simulink model "HardwareInteg_draft2"  (R2023a)
settings: Solver=VariableStepAuto  StartTime=0.0  StopTime=inf  FixedStep=0.01  RelTol=1e-3
model workspace (MAT data in the model file):
  D = 0
  I = 0
  N = 100
  P = 1
  setpoint = 1
undefined symbols (not defined in the file or in its folder): daq
libraries: simulink x4, dspstat3 x3, daqlib x2, slpidlib x2, checkpacklib x1, spsTriangleGeneratorLib x1
settings Model: Creator=Siril TD  LastModifiedBy=Siril TD
settings OptimizationCC: DefaultParameterBehavior=Inlined  EnhancedBackFolding=on  PassReuseOutputArgsThreshold=0  OptimizeBlockOrder=speed  DifferentSizesBufferReuse=on
settings DebuggingCC: ParameterTunabilityLossMsg=error
settings HardwareCC: TargetBitPerPointer=64  TargetBitPerSizeT=64  TargetBitPerPtrDiffT=64  TargetLongLongMode=on  TargetIntDivRoundTo=Zero  TargetEndianess=LittleEndian  TargetWordSize=64  TargetHWDeviceType=MATLAB Host  ProdEqTarget=off
settings SFSimCC: SimGenImportedTypeDefs=on  SimTargetLang=C++
settings RTWCC: GenCodeOnly=on
settings CodeAppCC: ForceParamTrailComments=on  MaxIdLength=63  OperatorAnnotations=on

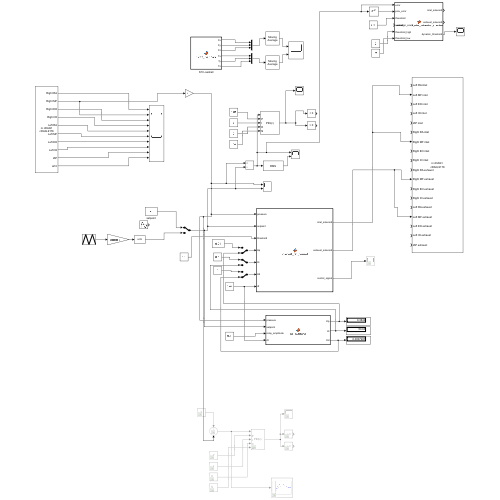
[thumbnail: Simulink's stored preview of the top-level diagram]
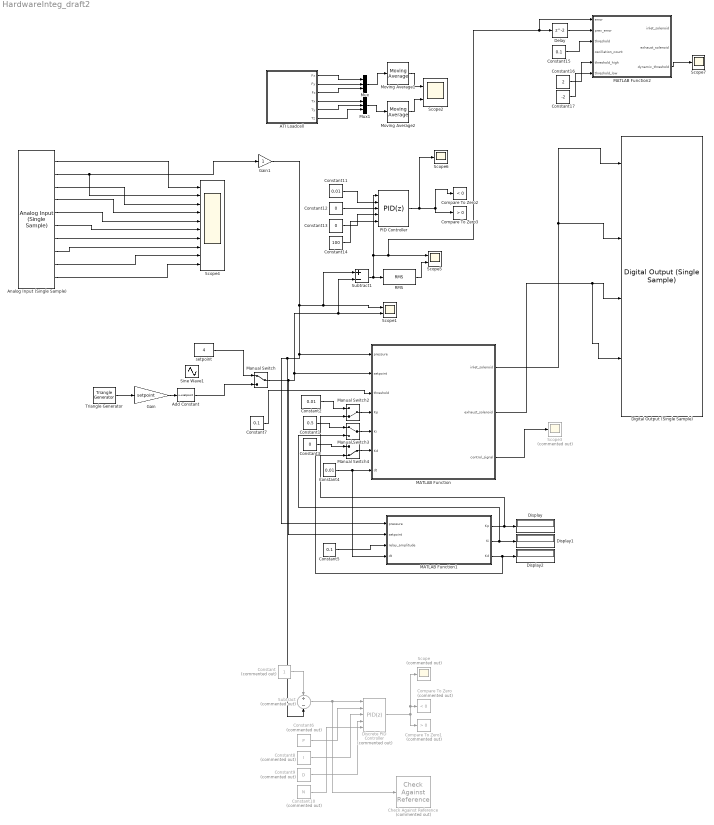
== system HardwareInteg_draft2 ==
  ATI Loadcell : MATLAB Function  TreatAsAtomicUnit=on
  Add Constant : Bias  Bias=setpoint  SaturateOnIntegerOverflow=off
  Analog Input (Single Sample) : daqlib/Analog Input (Single Sample)  DeviceMenu=ni cDAQ1 (cDAQ-9178)  Device=ni cDAQ1 (cDAQ-9178)  ModuleInfo=cDAQ1Mod1(NI 9205)  ObjConstructor=daq.createSession('ni')  BlockSampleTime=0.001  NChannelsSelected=10  Channels=0$ai0$$cDAQ1Mod1$1$4$1$1$#1$ai1$Right RA$cDAQ1Mod1$1$4$1$1$#1$ai2$Right MF$cDAQ1Mod1$1$4$1$1$#1$ai3$Right EO$cDAQ1Mod1$1$4$1$1$#1$ai4$Right IO$cDAQ1Mod1$1$4$1$1$#1$ai5$Left RA$cDAQ1Mod1$1$4$1$1$#1$ai6$Left MF$cDAQ1Mod1$1$4$1$1$#1$ai7$Left EO$cDAQ1Mod1$1$4$1$1$#1$ai8$Left IO$cDAQ1Mod1$1$4$1$1$#1$ai9$IAP$cDAQ1Mod1$1$4$1$1$#1$ai10$$cDAQ1Mod1$1$4$1$1$#0$ai11$$cDAQ1Mod1$1$4$1$1$#0$ai12$$cDAQ1Mod1$1$4$1$1$#0$ai13$$cDAQ1Mod1$1$4$1$1$#0$ai14$$cDAQ1Mod1$1$4$1$1$#0$ai15$$cDAQ1Mod1$1$4$1$1$#0$ai16$$cDAQ1Mod1$1$4$3$1$#0$ai17$$cDAQ1Mod1$1$4$3$1$#0$ai18$$cDAQ1Mod1$1$4$3$1$#0$ai19$$cDAQ1Mod1$1$4$3$1$#0$ai20$$cDAQ1Mod1$1$4$3$1$#0$ai21$$cDAQ1Mod1$1$4$3$1$#0$ai22$$cDAQ1Mod1$1$4$3$1$#0$ai23$$cDAQ1Mod1$1$4$3$1$#0$ai24$$cDAQ1Mod1$1$4$1$1$#0$ai25$$cDAQ1Mod1$1$4$1$1$#0$ai26$$cDAQ1Mod1$1$4$1$1$#0$ai27$$cDAQ1Mod1$1$4$1$1$#0$ai28$$cDAQ1Mod1$1$4$1$1$#0$ai29$$cDAQ1Mod1$1$4$1$1$#0$ai30$$cDAQ1Mod1$1$4$1$1$#0$ai31$$cDAQ1Mod1$1$4$1$1$#  NPorts=1 per channel  OutputTimestamp=off
  Check Against Reference : checkpacklib/Check Against Reference  Commented=on  InstantiateOnLoad=on  enabled=on  stopWhenAssertionFail=off  export=off  ViewDlgPos=[100 200 510 390]  OpenViewOnLoad=off  LaunchViewOnOpen=on  TimeUnits=seconds  EnableReferenceBound=on  AbsTolerance=0  RelTolerance=0.01  ReferenceTimes=[0 10]  ReferenceAmplitudes=[0 0]
      settings: LibrarySourceBlock=sdolib/Signal Constraints/Check Against Reference
  Compare To Zero : simulink/Logic and Bit Operations/Compare To Zero  Commented=on  relop=<  OutDataTypeStr=boolean
  Compare To Zero1 : simulink/Logic and Bit Operations/Compare To Zero  Commented=on  relop=>  OutDataTypeStr=boolean
  Compare To Zero2 : simulink/Logic and Bit Operations/Compare To Zero  relop=<  OutDataTypeStr=boolean
  Compare To Zero3 : simulink/Logic and Bit Operations/Compare To Zero  relop=>  OutDataTypeStr=boolean
  Constant : Constant  Commented=on
  Constant1 : Constant  Value=0.5
  Constant10 : Constant  Commented=on  Value=N
  Constant11 : Constant  Value=0.01
  Constant12 : Constant  Value=0
  Constant13 : Constant  Value=0
  Constant14 : Constant  Value=100
  Constant15 : Constant  Value=0.1
  Constant16 : Constant  Value=2
  Constant17 : Constant  Value=-2
  Constant2 : Constant  Value=0.01
  Constant3 : Constant  Value=0
  Constant4 : Constant  Value=0.01
  Constant5 : Constant  Value=0.1
  Constant6 : Constant  Commented=on  Value=P
  Constant7 : Constant  Value=0.1
  Constant8 : Constant  Commented=on  Value=I
  Constant9 : Constant  Commented=on  Value=D
  Delay : Delay
  Digital Output (Single Sample) : daqlib/Digital Output (Single Sample)  DeviceMenu=ni cDAQ1 (cDAQ-9178)  Device=ni cDAQ1 (cDAQ-9178)  ModuleInfo=cDAQ1Mod3(NI 9485)cDAQ1Mod4(NI 9485)cDAQ1Mod5(NI 9485)cDAQ1Mod6(NI 9485)  ObjConstructor=daq.createSession('ni')  BlockSampleTime=0.001  IsDigitalInput=off  NLinesSelected=18  Lines=0$port0/line0$$cDAQ1Mod3$#1$port0/line1$Left RA inlet$cDAQ1Mod3$#1$port0/line2$Left MF inlet$cDAQ1Mod3$#1$port0/line3$Left EO inlet$cDAQ1Mod3$#1$port0/line4$Left IO inlet$cDAQ1Mod3$#1$port0/line5$IAP inlet$cDAQ1Mod3$#0$port0/line6$$cDAQ1Mod3$#0$port0/line7$$cDAQ1Mod3$#0$port0/line0$$cDAQ1Mod4$#1$port0/line1$Right RA inlet$cDAQ1Mod4$#0$port0/line2$$cDAQ1Mod4$#1$port0/line3$Right MF inlet$cDAQ1Mod4$#0$port0/line4$$cDAQ1Mod4$#1$port0/line5$Right EO inlet$cDAQ1Mod4$#1$port0/line6$Right IO inlet$cDAQ1Mod4$#0$port0/line7$$cDAQ1Mod4$#0$port0/line0$$cDAQ1Mod5$#1$port0/line1$Right RA exhaust$cDAQ1Mod5$#0$port0/line2$$cDAQ1Mod5$#1$port0/line3$Right MF exhaust$cDAQ1Mod5$#0$port0/line4$$cDAQ1Mod5$#1$port0/line5$Right EO exhaust$cDAQ1Mod5$#1$port0/line6$Right IO exhaust$cDAQ1Mod5$#0$port0/line7$$cDAQ1Mod5$#0$port0/line0$$cDAQ1Mod6$#1$port0/line1$Left RA exhaust$cDAQ1Mod6$#1$port0/line2$Left MF exhaust$cDAQ1Mod6$#1$port0/line3$Left EO exhaust$cDAQ1Mod6$#1$port0/line4$Left IO exhaust$cDAQ1Mod6$#1$port0/line5$IAP exhaust$cDAQ1Mod6$#0$port0/line6$$cDAQ1Mod6$#0$port0/line7$$cDAQ1Mod6$#  NPorts=1 per line
  Discrete PID Controller : slpidlib/PID Controller  Commented=on  Controller=PID  Form=Parallel  TimeDomain=Discrete-time  UseExternalTs=off  SampleTime=0.01  IntegratorMethod=Forward Euler  FilterMethod=Forward Euler  ControllerParametersSource=external  P=0  I=-100  UseKiTs=off  D=0  N=100  UseFilter=on  TunerSelectOption=Transfer Function Based (PID Tuner App)  InitialConditionSource=internal  InitialConditionForIntegrator=0  InitialConditionForFilter=0  DifferentiatorICPrevScaledInput=0  ExternalReset=none  TrackingMode=off  Kt=1  LimitOutput=off  SatLimitsSource=internal  UpperSaturationLimit=inf  LowerSaturationLimit=-inf  LinearizeAsGain=off  AntiWindupMode=none  Kb=1  LimitIntegrator=off  UpperIntegratorSaturationLimit=inf  LowerIntegratorSaturationLimit=-inf  POutMin=[]  POutMax=[]  IOutMin=[]  IOutMax=[]  DOutMin=[]  DOutMax=[]  NOutMin=[]  NOutMax=[]  SumOutMin=[]  SumOutMax=[]  SaturationOutMin=[]  SaturationOutMax=[]  PParamMin=[]  PParamMax=[]  IParamMin=[]  IParamMax=[]  DParamMin=[]  DParamMax=[]  NParamMin=[]  NParamMax=[]  KbParamMin=[]  KbParamMax=[]  KtParamMin=[]  KtParamMax=[]  KbOutMin=[]  KbOutMax=[]  KtOutMin=[]  KtOutMax=[]  IntegratorOutMin=[]  IntegratorOutMax=[]  FilterOutMin=[]  FilterOutMax=[]  SumI1OutMin=[]  SumI1OutMax=[]  SumI2OutMin=[]  SumI2OutMax=[]  SumI3OutMin=[]  SumI3OutMax=[]  SumI4OutMin=[]  SumI4OutMax=[]  SumDOutMin=[]  SumDOutMax=[]  DifferentiatorOutMin=[]  DifferentiatorOutMax=[]  FilterDiffOutCoefMin=[]  FilterDiffOutCoefMax=[]  ReciprocalOutMin=[]  ReciprocalOutMax=[]  SumDenOutMin=[]  SumDenOutMax=[]  SumNumOutMin=[]  SumNumOutMax=[]  DivideOutMin=[]  DivideOutMax=[]  UdiffTsProdOutMin=[]  UdiffTsProdOutMax=[]  NTsProdOutMin=[]  NTsProdOutMax=[]  UintegralTsProdOutMin=[]  UintegralTsProdOutMax=[]  UngainTsProdOutMin=[]  UngainTsProdOutMax=[]  ClampingZeroOutDataTypeStr=Inherit: Inherit via back propagation  ClampingZeroOutMin=[]  ClampingZeroOutMax=[]  FilterDenConstantOutDataTypeStr=Inherit: Inherit via back propagation  FilterDenConstantOutMin=[]  FilterDenConstantOutMax=[]  PCopyOutDataTypeStr=Inherit: Inherit via back propagation  PCopyOutMin=[]  PCopyOutMax=[]  NCopyOutDataTypeStr=Inherit: Inherit via back propagation  NCopyOutMin=[]  NCopyOutMax=[]  IntegratorContinuousStateAttributes=''  IntegratorStateMustResolveToSignalObject=off  IntegratorRTWStateStorageClass=Auto  FilterContinuousStateAttributes=''  FilterStateMustResolveToSignalObject=off  FilterRTWStateStorageClass=Auto  ParallelPVariant=ExternalParameters  IdealPVariant=Disabled  IVariant=ExternalParameters  DVariant=ExternalParameters  IntegratorVariant=Discrete  SatVariant=Disabled  AWVariant=Passthrough  PCopyVariant=Disabled  TRVariant=Disabled  FdbkBlocksVariant=Forward  IdealPFdbkVariant=Disabled  SatFdbkVariant=Disabled  DerivativeFilterVariant=ForwardEulerFilter  NVariant=ExternalParameters  NCopyVariant=Disabled  FilterICVariant=InternalICsFilter  IntegratorICVariant=InternalICs  ExternalResetVariant=Disabled  TRSumVariant=Passthrough  SumFdbkVariant=Disabled  SumVariant=Sum_PID  TsampFilterVariant=InternalTs  TsampNgainVariant=Passthrough  TsampIntegralVariant=Disabled_SignalSpec  ExternalSaturationOutDataTypeStr=Inherit: Same as second input
      settings: LibrarySourceBlock=simulink/Discrete/Discrete PID Controller
  Display : Display
  Display1 : Display
  Display2 : Display
  Gain : Gain  Gain=setpoint
  Gain1 : Gain
  MATLAB Function : MATLAB Function  TreatAsAtomicUnit=on
  MATLAB Function1 : MATLAB Function  TreatAsAtomicUnit=on
  MATLAB Function2 : MATLAB Function  TreatAsAtomicUnit=on
  Manual Switch : ManualSwitch
  Manual Switch2 : ManualSwitch  CurrentSetting=0
  Manual Switch3 : ManualSwitch
  Manual Switch4 : ManualSwitch  CurrentSetting=0
  Moving Average1 : dspstat3/Moving Average  Method=Sliding window  ForgettingFactorPort=off  SpecifyWindowLength=on  WindowLength=4  OverlapLength=3  AllowArbitraryInputLength=off  ForgettingFactor=0.9  SimulateUsing=Code generation
  Moving Average2 : dspstat3/Moving Average  Method=Sliding window  ForgettingFactorPort=off  SpecifyWindowLength=on  WindowLength=4  OverlapLength=3  AllowArbitraryInputLength=off  ForgettingFactor=0.9  SimulateUsing=Code generation
  Mux : Mux  Inputs=3
  Mux1 : Mux  Inputs=3
  PID Controller : slpidlib/PID Controller  Controller=PID  Form=Parallel  TimeDomain=Discrete-time  UseExternalTs=off  SampleTime=-1  IntegratorMethod=Forward Euler  FilterMethod=Forward Euler  ControllerParametersSource=external  P=1  I=1  UseKiTs=off  D=0  N=100  UseFilter=on  TunerSelectOption=Transfer Function Based (PID Tuner App)  InitialConditionSource=internal  InitialConditionForIntegrator=0  InitialConditionForFilter=0  DifferentiatorICPrevScaledInput=0  ExternalReset=none  TrackingMode=off  Kt=1  LimitOutput=off  SatLimitsSource=internal  UpperSaturationLimit=inf  LowerSaturationLimit=-inf  LinearizeAsGain=on  AntiWindupMode=none  Kb=1  LimitIntegrator=off  UpperIntegratorSaturationLimit=inf  LowerIntegratorSaturationLimit=-inf  POutMin=[]  POutMax=[]  IOutMin=[]  IOutMax=[]  DOutMin=[]  DOutMax=[]  NOutMin=[]  NOutMax=[]  SumOutMin=[]  SumOutMax=[]  SaturationOutMin=[]  SaturationOutMax=[]  PParamMin=[]  PParamMax=[]  IParamMin=[]  IParamMax=[]  DParamMin=[]  DParamMax=[]  NParamMin=[]  NParamMax=[]  KbParamMin=[]  KbParamMax=[]  KtParamMin=[]  KtParamMax=[]  KbOutMin=[]  KbOutMax=[]  KtOutMin=[]  KtOutMax=[]  IntegratorOutMin=[]  IntegratorOutMax=[]  FilterOutMin=[]  FilterOutMax=[]  SumI1OutMin=[]  SumI1OutMax=[]  SumI2OutMin=[]  SumI2OutMax=[]  SumI3OutMin=[]  SumI3OutMax=[]  SumI4OutMin=[]  SumI4OutMax=[]  SumDOutMin=[]  SumDOutMax=[]  DifferentiatorOutMin=[]  DifferentiatorOutMax=[]  FilterDiffOutCoefMin=[]  FilterDiffOutCoefMax=[]  ReciprocalOutMin=[]  ReciprocalOutMax=[]  SumDenOutMin=[]  SumDenOutMax=[]  SumNumOutMin=[]  SumNumOutMax=[]  DivideOutMin=[]  DivideOutMax=[]  UdiffTsProdOutMin=[]  UdiffTsProdOutMax=[]  NTsProdOutMin=[]  NTsProdOutMax=[]  UintegralTsProdOutMin=[]  UintegralTsProdOutMax=[]  UngainTsProdOutMin=[]  UngainTsProdOutMax=[]  ClampingZeroOutDataTypeStr=Inherit: Inherit via back propagation  ClampingZeroOutMin=[]  ClampingZeroOutMax=[]  FilterDenConstantOutDataTypeStr=Inherit: Inherit via back propagation  FilterDenConstantOutMin=[]  FilterDenConstantOutMax=[]  PCopyOutDataTypeStr=Inherit: Inherit via back propagation  PCopyOutMin=[]  PCopyOutMax=[]  NCopyOutDataTypeStr=Inherit: Inherit via back propagation  NCopyOutMin=[]  NCopyOutMax=[]  IntegratorContinuousStateAttributes=''  IntegratorStateMustResolveToSignalObject=off  IntegratorRTWStateStorageClass=Auto  FilterContinuousStateAttributes=''  FilterStateMustResolveToSignalObject=off  FilterRTWStateStorageClass=Auto  ParallelPVariant=ExternalParameters  IdealPVariant=Disabled  IVariant=ExternalParameters  DVariant=ExternalParameters  IntegratorVariant=Discrete  SatVariant=Disabled  AWVariant=Passthrough  PCopyVariant=Disabled  TRVariant=Disabled  FdbkBlocksVariant=Forward  IdealPFdbkVariant=Disabled  SatFdbkVariant=Disabled  DerivativeFilterVariant=ForwardEulerFilter  NVariant=ExternalParameters  NCopyVariant=Disabled  FilterICVariant=InternalICsFilter  IntegratorICVariant=InternalICs  ExternalResetVariant=Disabled  TRSumVariant=Passthrough  SumFdbkVariant=Disabled  SumVariant=Sum_PID  TsampFilterVariant=InternalTs  TsampNgainVariant=Passthrough  TsampIntegralVariant=Disabled_SignalSpec  ExternalSaturationOutDataTypeStr=Inherit: Same as second input
  RMS : dspstat3/RMS  run=off  directionMode=Each column  dimension=1  InputProcessing=Columns as channels (frame based)  reset_popup=None
  Scope : Scope  Commented=on
  Scope1 : Scope  NumInputPorts=2
  Scope2 : Scope  NumInputPorts=2
  Scope3 : Scope  Commented=on
  Scope4 : Scope  NumInputPorts=10
  Scope5 : Scope  NumInputPorts=2
  Scope6 : Scope
  Scope7 : Scope
  Sine Wave1 : Sin  Amplitude=2  Bias=3  Frequency=0.005  SampleTime=0
  Subtract : Sum  Commented=on  Inputs=+-
  Subtract1 : Sum  Inputs=+-
  Triangle Generator : spsTriangleGeneratorLib/Triangle Generator  Freq=1  Phase=0  Ts=0
  setpoint : Constant  Value=4
  wires:
  Analog Input (Single Sample)/1 -> Scope4/1
  Constant4/1 -> MATLAB Function1/4(dt), MATLAB Function/7(dt)
  MATLAB Function/3(control_signal) -> Scope3/1
  Constant5/1 -> MATLAB Function1/3(relay_amplitude)
  MATLAB Function1/2(Ki) -> Manual Switch3/2, Display1/1
  MATLAB Function1/3(Kd) -> Manual Switch4/2, Display2/1
  Manual Switch/1 -> Subtract1/2, Scope1/2, MATLAB Function/2(setpoint), MATLAB Function1/2(setpoint)
  Constant7/1 -> MATLAB Function/3(threshold)
  ATI Loadcell/1(Fx) -> Mux/1
  ATI Loadcell/2(Fy) -> Mux/2
  ATI Loadcell/3(Fz) -> Mux/3
  ATI Loadcell/4(Tx) -> Mux1/1
  ATI Loadcell/5(Ty) -> Mux1/2
  ATI Loadcell/6(Tz) -> Mux1/3
  Mux/1 -> Moving Average1/1
  Moving Average1/1 -> Scope2/1
  Mux1/1 -> Moving Average2/1
  Moving Average2/1 -> Scope2/2
  Analog Input (Single Sample)/3 -> Scope4/3
  Analog Input (Single Sample)/4 -> Scope4/4
  Analog Input (Single Sample)/5 -> Scope4/5
  Analog Input (Single Sample)/6 -> Scope4/6
  Analog Input (Single Sample)/7 -> Scope4/7
  Analog Input (Single Sample)/8 -> Scope4/8
  Analog Input (Single Sample)/9 -> Scope4/9
  Analog Input (Single Sample)/10 -> Scope4/10
  MATLAB Function1/1(Kp) -> Manual Switch2/2, Display/1
  Subtract/1 -> Check Against Reference/1, Discrete PID Controller/1
  Discrete PID Controller/1 -> Scope/1, Compare To Zero/1, Compare To Zero1/1
  Constant/1 -> Subtract/1
  Constant6/1 -> Discrete PID Controller/2
  Constant8/1 -> Discrete PID Controller/3
  Constant9/1 -> Discrete PID Controller/4
  Constant10/1 -> Discrete PID Controller/5
  Manual Switch2/1 -> MATLAB Function/4(Kp)
  Manual Switch4/1 -> MATLAB Function/6(Kd)
  Manual Switch3/1 -> MATLAB Function/5(Ki)
  Constant2/1 -> Manual Switch2/1
  Constant1/1 -> Manual Switch3/1
  Constant3/1 -> Manual Switch4/1
  Subtract1/1 -> RMS/1, MATLAB Function2/1(error), Delay/1, Scope5/1, PID Controller/1
  RMS/1 -> Scope5/2
  Triangle Generator/1 -> Gain/1
  Gain/1 -> Add Constant/1
  Add Constant/1 -> Manual Switch/2
  setpoint/1 -> Manual Switch/1
  PID Controller/1 -> Scope6/1, Compare To Zero2/1, Compare To Zero3/1
  Constant11/1 -> PID Controller/2
  Constant12/1 -> PID Controller/3
  Constant13/1 -> PID Controller/4
  Constant14/1 -> PID Controller/5
  Delay/1 -> MATLAB Function2/2(prev_error)
  Constant15/1 -> MATLAB Function2/3(threshold)
  MATLAB Function2/3(dynamic_threshold) -> Scope7/1
  Constant16/1 -> MATLAB Function2/5(threshold_high)
  Constant17/1 -> MATLAB Function2/6(threshold_low)
  MATLAB Function/1(inlet_solenoid) -> Digital Output (Single Sample)/7, Digital Output (Single Sample)/2
  MATLAB Function/2(exhaust_solenoid) -> Digital Output (Single Sample)/15, Digital Output (Single Sample)/11
  Gain1/1 -> MATLAB Function1/1(pressure), Subtract/2, MATLAB Function/1(pressure), Subtract1/1, Scope1/1
  Analog Input (Single Sample)/2 -> Gain1/1, Scope4/2

== matlab function HardwareInteg_draft2/MATLAB Function1 ==
  settings: updateMethod=DISCRETE
  data: pressure input; Kp output; setpoint input; relay_amplitude input; dt input; Ki output; Kd output
function [Kp, Ki, Kd] = pid_autotune(pressure, setpoint, relay_amplitude, dt)
    persistent error_prev relay_state oscillation_data time;


    kp = 0.03;
    ki = 0;
    kd = 0;


    % Initialize persistent variables
    if isempty(error_prev)
        error_prev = 0;
        relay_state = 1; % Start with positive relay state
        oscillation_data = [];
        time = 0;
    end

    % Calculate error
    error = setpoint - pressure;

    % Relay control logic
    if relay_state == 1 && error < relay_amplitude
        relay_state = -1;
        oscillation_data = [oscillation_data; time, pressure]; % Record time and response
    elseif relay_state == -1 && error > -relay_amplitude
        relay_state = 1;
        oscillation_data = [oscillation_data; time, pressure];
    end

    % Update time
    time = time + dt;

    % Once sufficient oscillation data is collected, compute PID gains
    if size(oscillation_data, 1) > 4
        % Calculate ultimate gain (Ku) and period (Tu)
        Ku = (4 * relay_amplitude) / (pi * std(diff(oscillation_data(:, 2))));
        Tu = mean(diff(oscillation_data(:, 1)));

        % Compute PID gains using Ziegler-Nichols tuning rules
        Kp = 0.6 * Ku;
        Ki = 1.2 * Ku / Tu;
        Kd = 0.075 * Ku * Tu;

        return; % Exit function with updated gains
    else
        Kp = 0.05; Ki = 0; Kd = 0; % Gains not ready
    end
end




% function [Kp, Ki, Kd] = pid_autotune(pressure, setpoint, relay_amplitude, dt)
%     persistent error_prev relay_state oscillation_data time last_switch_time filtered_pressure;
% 
% 
%     % Low-pass filter coefficient (adjust for smoother response)
%     alpha = 0.2; % 0.1 - 0.3 for strong filtering, 0.6 - 0.9 for weak filtering
% 
%      kp = 0.03;
%      ki = 0;
%      kd = 0;
% 
%     % Initialize persistent variables
%     if isempty(error_prev)
%         error_prev = 0;
%         relay_state = 1;
%         oscillation_data = [];
%         time = 0;
%         last_switch_time = 0;
%         filtered_pressure = pressure; % Initialize filtered pressure
%     end
% 
%     % Apply Low-Pass Filter to smooth sensor data
%     filtered_pressure = alpha * pressure + (1 - alpha) * filtered_pressure;
% 
%     % Compute error using filtered pressure
%     error = setpoint - filtered_pressure;
% 
%     % Adaptive relay amplitude (prevents excessive switching near setpoint)
%     relay_amplitude = max(0.1, 0.2 * abs(setpoint - filtered_pressure));
% 
%     % Delay before switching states (prevents chattering)
%     switch_delay = 0.1; % 100ms minimum switching delay
%     if (relay_state == 1 && error < relay_amplitude) && (time - last_switch_time > switch_delay)
%         relay_state = -1;
%         last_switch_time = time;
%         oscillation_data = [oscillation_data; time, filtered_pressure];
%     elseif (relay_state == -1 && error > -relay_amplitude) && (time - last_switch_time > switch_delay)
%         relay_state = 1;
%         last_switch_time = time;
%         oscillation_data = [oscillation_data; time, filtered_pressure];
%     end
% 
%     % Update time
%     time = time + dt;
% 
%     % Once sufficient oscillation data is collected, compute PID gains
%     if size(oscillation_data, 1) > 4
%         % Calculate ultimate gain (Ku) and period (Tu)
%         Ku = (4 * relay_amplitude) / (pi * std(diff(oscillation_data(:, 2))));
%         Tu = mean(diff(oscillation_data(:, 1)));
% 
%         % Adjust PID tuning rules for smoother response
%         Kp = 0.6 * Ku;      % Standard Z-N tuning
%         Ki = 0.3 * Ku / Tu; % Reduced Ki to prevent chatter
%         Kd = 0.075 * Ku * Tu; % Standard Z-N derivative tuning
% 
%         % Limit Ki to prevent integral windup
%         Ki = min(Ki, 0.5);
% 
%         return;
%     else
%         Kp = 0.05; Ki = 0; Kd = 0; % Gains not ready
%     end
% end

== matlab function HardwareInteg_draft2/MATLAB Function ==
  settings: updateMethod=DISCRETE
  data: pressure input; setpoint input; threshold input; Kp input; Ki input; Kd input; inlet_solenoid output; exhaust_solenoid output; control_signal output; dt input
% function [inlet_solenoid, exhaust_solenoid] = solenoid_control(error, threshold)
%     % Initialize outputs as boolean (false = 0, true = 1)
%     inlet_solenoid = false;  % Default: OFF
%     exhaust_solenoid = false; % Default: OFF
% 
%     % Inlet solenoid control (turn on if pressure is too low)
%     if error > threshold
%         inlet_solenoid = true;  % Turn ON inlet solenoid
%     end
% 
%     % Exhaust solenoid control (turn on if pressure is too high)
%     if error < -threshold
%         exhaust_solenoid = true;  % Turn ON exhaust solenoid
%     end
% end


% function [inlet_solenoid, exhaust_solenoid, dynamic_threshold] = solenoid_control_with_adaptive_threshold(error, prev_error, threshold, oscillation_count, threshold_high, threshold_low)
%     % Define thresholds
%     dynamic_threshold = threshold;  % Default threshold
%     inlet_solenoid = false;         % Default: OFF
%     exhaust_solenoid = false;       % Default: OFF
% 
%     % Oscillation detection logic:
%     % Check if the error changes direction (from positive to negative or vice versa)
%     if (error > 0 && prev_error < 0) || (error < 0 && prev_error > 0)
%         oscillation_count = oscillation_count + 1;  % Increase oscillation count if direction changes
%     else
%         oscillation_count = 0;  % Reset if no direction change
%     end
% 
%     % Adjust threshold based on oscillation count:
%     if oscillation_count > 3  % You can adjust this threshold for detection sensitivity
%         dynamic_threshold = threshold_high;  % Set higher threshold to reduce switching
%     elseif abs(error) < 0.05  % If error is small (close to setpoint), reduce the threshold to 0.1
%         dynamic_threshold = threshold_low;
%     end
% 
%     % Solenoid control based on the dynamic threshold:
%     if error > dynamic_threshold
%         inlet_solenoid = true;  % Turn ON inlet solenoid if error is large and positive
%     elseif error < -dynamic_threshold
%         exhaust_solenoid = true;  % Turn ON exhaust solenoid if error is large and negative
%     else
%         inlet_solenoid = false;  % Keep OFF if error is within deadband
%         exhaust_solenoid = false;  % Keep OFF if error is within deadband
%     end
% 
%     % Output the adjusted dynamic threshold for monitoring or debugging
% end




function [inlet_solenoid, exhaust_solenoid,control_signal] = solenoid_pid_control(pressure, setpoint, threshold, Kp, Ki, Kd, dt)
    % Persistent variables to maintain state between function calls
    persistent integral_error prev_error;

    % Initialize persistent variables on first run
    if isempty(integral_error)
        integral_error = 0;
    end
    if isempty(prev_error)
        prev_error = 0;
    end

  % Set default PID gains if they are not provided
    if isempty(Kp)
        Kp = 1;  % Default proportional gain
    end
    if isempty(Ki)
        Ki = 0.1;  % Default integral gain
    end
    if isempty(Kd)
        Kd = 0.0;  % Default derivative gain
    end


    % Calculate error
    error = setpoint - pressure;

    % Apply low-pass filter to the error
    alpha = 1;
    filtered_error = 0;
    filtered_error = alpha * error + (1 - alpha) * filtered_error;  % Simple low-pass filter


    % Update integral and derivative components
    integral_error = integral_error + error * dt; % Accumulated error
    derivative_error = (error - prev_error) / dt; % Rate of change of error

    % PID control output
    control_signal = Kp * error + Ki * integral_error + Kd * derivative_error;

    % Set thresholds for valve control
   % threshold = 0.1; % Adjust this as needed for your system

    % Valve logic based on control signal
    inlet_solenoid = false;  % Default: OFF
    exhaust_solenoid = false; % Default: OFF

    if control_signal > threshold
        inlet_solenoid = true;  % Open inlet valve
    elseif control_signal < -threshold
        exhaust_solenoid = true;  % Open exhaust valve
    end

    % Update previous error for the next derivative calculation
    prev_error = error;
end

== matlab function HardwareInteg_draft2/MATLAB Function2 ==
  data: error input; inlet_solenoid output; prev_error input; threshold input; oscillation_count input; threshold_high input; threshold_low input; exhaust_solenoid output; dynamic_threshold output
function [inlet_solenoid, exhaust_solenoid, dynamic_threshold] = solenoid_control_with_adaptive_threshold(error, prev_error, threshold, oscillation_count, threshold_high, threshold_low)
    % Define thresholds
    dynamic_threshold = threshold;  % Default threshold
    inlet_solenoid = false;         % Default: OFF
    exhaust_solenoid = false;       % Default: OFF

    % Oscillation detection logic:
    % Check if the error changes direction (from positive to negative or vice versa)
    if (error > 0 && prev_error < 0) || (error < 0 && prev_error > 0)
        oscillation_count = oscillation_count + 1;  % Increase oscillation count if direction changes
    else
        oscillation_count = 0;  % Reset if no direction change
    end

    % Adjust threshold based on oscillation count:
    if oscillation_count > 3  % You can adjust this threshold for detection sensitivity
        dynamic_threshold = threshold_high;  % Set higher threshold to reduce switching
    elseif abs(error) < 0.05  % If error is small (close to setpoint), reduce the threshold to 0.1
        dynamic_threshold = threshold_low;
    end

    % Solenoid control based on the dynamic threshold:
    if error < -dynamic_threshold
        inlet_solenoid = true;  % Turn ON inlet solenoid if error is large and positive
    elseif error > dynamic_threshold
        exhaust_solenoid = true;  % Turn ON exhaust solenoid if error is large and negative
    else
        inlet_solenoid = false;  % Keep OFF if error is within deadband
        exhaust_solenoid = false;  % Keep OFF if error is within deadband
    end

    % Output the adjusted dynamic threshold for monitoring or debugging
end

== matlab function HardwareInteg_draft2/ATI Loadcell ==
  data: Fx output; Fy output; Fz output; Tx output; Ty output; Tz output
function [Fx, Fy, Fz, Tx, Ty, Tz] = netFT_readData()
    % Declare the extrinsic wrapper function
    coder.extrinsic('ATI_Wrapper');  % Tell Simulink that myWrapper is an external function

    % Initialize output variables as numeric types
    Fx = 0;
    Fy = 0;
    Fz = 0;
    Tx = 0;
    Ty = 0;
    Tz = 0;

    % Call the wrapper function
    [Fx, Fy, Fz, Tx, Ty, Tz] = ATI_Wrapper();  % Get the force and torque data
end
